simulink model "ChirpTest_ExC"  (R2021b)
settings: Solver=VariableStepAuto  StartTime=0.0  StopTime=30.0  RelTol=1e-3
values from neighbouring files (symbols this model uses):
  Asfo = A - L*C    [ControllerDesign.m]
  Bsfo = [B-(L*D), L]    [ControllerDesign.m]
  Csfo = K    [ControllerDesign.m]
  Dsfo = zeros(1,3)    [ControllerDesign.m]
settings Model: Creator=westwick  LastModifiedBy=Andrey
settings SolverCC: AlgebraicLoopSolver=TrustRegion
settings DebuggingCC: SFMachineParentedDataDiag=warning
settings SFSimCC: CustomCodeUndefinedFunction=UseInterfaceOnly

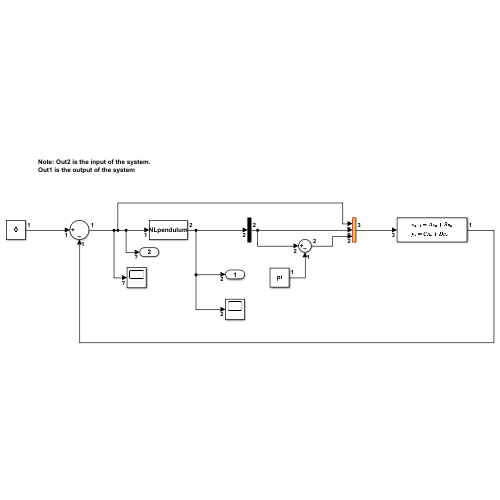
[thumbnail: Simulink's stored preview of the top-level diagram]
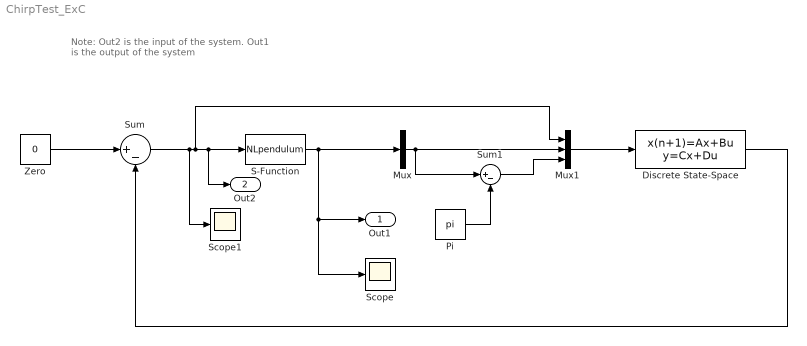
== system ChirpTest_ExC ==
  note: Note: Out2 is the input of the system.
      | Out1 is the output of the system
  Discrete State-Space : DiscreteStateSpace  A=Asfo  B=Bsfo  C=Csfo  D=Dsfo  InitialCondition=0.25  SampleTime=1/200
  Mux : Mux  Inputs=1
  Mux1 : Mux  Inputs=3
  Pi : Constant  Value=pi  OutDataTypeStr=Inherit: Inherit via back propagation
  S-Function : S-Function  FunctionName=NLpendulum  SFunctionDeploymentMode=off  EnableBusSupport=off
  Scope : Scope
  Scope1 : Scope
  Sum : Sum  Inputs=|+-
  Sum1 : Sum  Inputs=|+-
  Zero : Constant  Value=0  OutDataTypeStr=Inherit: Inherit via back propagation  SampleTime=1/200
  Out1 : Outport  VectorParamsAs1DForOutWhenUnconnected=off
  Out2 : Outport  Port=2  VectorParamsAs1DForOutWhenUnconnected=off
  wires:
  Sum/1 -> Scope1/1, Mux1/1, S-Function/1, Out2/1
  Zero/1 -> Sum/1
  S-Function/1 -> Mux/1, Out1/1, Scope/1
  Discrete State-Space/1 -> Sum/2
  Mux/1 -> Sum1/1, Mux1/2
  Sum1/1 -> Mux1/3
  Pi/1 -> Sum1/2
  Mux1/1 -> Discrete State-Space/1
